simulink model "sim_file"  (R2018b)
settings: Solver=VariableStepAuto  StartTime=0.0  StopTime=10.0  RelTol=1e-3
values from neighbouring files (symbols this model uses):
  A = eval(A_eq)    [main_cntl.m]    (also in main_sys.m)
  B = eval(B_eq)    [main_cntl.m]    (also in main_sys.m)
  C = [ 0 , 1  , 0  ,  0 ,  0  ,  0 , 0 ... (first row only)    [main_sys.m]
  C_ctl = [0 0 114594.2 0.001 -114594.2 -0.001]    [cntl_sys.mat]    (also in main_cntl.m = [0 , 0  , Ks , ds , -Ks , -ds  ]; main_sys.m = C_ctl)
  D = 0    [main_sys.m]
  Rk = .5*diag(ones(1,2))    [main_sys.m]
  sys_sys = ss(A,B,C,0)    [main_sys.m]
undefined symbols (not defined in the file or in its folder): Continuous, Time
libraries: ctrlSharedLib x1
settings Model: Creator=eshojaei  LastModifiedBy=eshojaei

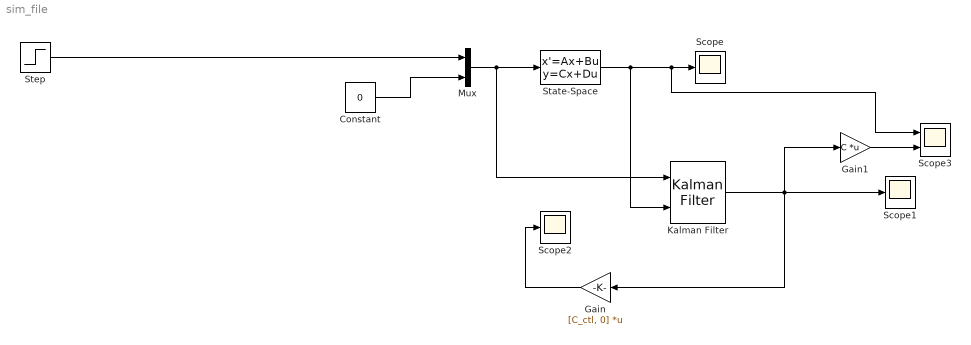
== system sim_file ==
  Constant : Constant  Value=0
  Gain : Gain  Gain=[C_ctl, 0]  Multiplication=Matrix(K*u)
  Gain1 : Gain  Gain=C  Multiplication=Matrix(K*u)
  Kalman Filter : ctrlSharedLib/Kalman Filter  TimeDomain=Continuous-Time  UseCurrentEstimator=off  ModelSource=LTI State-Space Variable  ModelSourceVariable=ss(A,B,C,D)  A=0.95  B=1  C=1  D=0  NumberOfStates=1  NumberOfInputs=1  NumberOfOutputs=1  InitialEstimateSource=Dialog  X0=0  P0=10  UseK=off  UseGH=off  NumberOfProcessNoiseInputs=1  G=1  TimeInvariantG=on  H=0  TimeInvariantH=on  Q=Qk  TimeInvariantQ=on  R=Rk  TimeInvariantR=on  N=0  TimeInvariantN=on  AddInputPort=on  AddEnablePort=off  OutputEstimatedY=off  OutputP=off  Ts=-1
      settings: SourceProductBaseCode=CT
  Mux : Mux  Inputs=2
  Scope : Scope
  Scope1 : Scope
  Scope2 : Scope
  Scope3 : Scope  NumInputPorts=2
  State-Space : StateSpace  A=sys_sys.A  B=sys_sys.B  C=sys_sys.C  D=sys_sys.D  InitialCondition=0
  Step : Step  Time=.1  After=5  SampleTime=0
  wires:
  Mux/1 -> Kalman Filter/1, State-Space/1
  Constant/1 -> Mux/2
  State-Space/1 -> Kalman Filter/2, Scope3/1, Scope/1
  Kalman Filter/1 -> Gain1/1, Gain/1, Scope1/1
  Gain/1 -> Scope2/1
  Step/1 -> Mux/1
  Gain1/1 -> Scope3/2
